simulink library "qrd_matrix_library"  (Simulink 8.7)
settings: Solver=ode45  StartTime=0.0  StopTime=10.0  RelTol=1e-3
values from neighbouring files (symbols this model uses):
  vectorization = 2    [qrd_test.m]
undefined symbols (not defined in the file or in its folder): AdvDSPBChannelOutDisplay, AdvDSPBDMemDisplay, Back_Substitution_instances, column_count, column_count_1, column_count_2, dpoly, dspba_ChannelInVis, dspba_ChannelOutVis, dspba_internal_get_channel_ports, evalAionMaskParam, latency, primtype, QRD_vectorization, recipsqrt, row, row_count, row_count_1, row_count_2, UseDontCare, value, x
libraries: DSPBAPrim x683, DSPBAControl x37, qrd_matrix_library x33, DSPBAVectorUtil x6, DSPBAVectorPrim x3
(part 3 of 8)

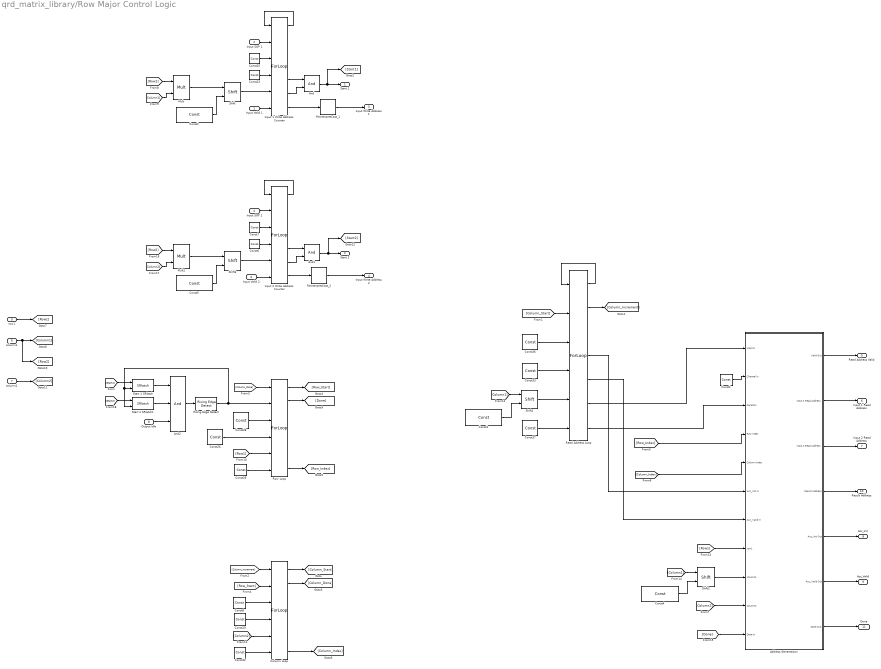
== system qrd_matrix_library/Row Major Control Logic ==
  Input Valid 1 : Inport
  Input SOP 1 : Inport  Port=2
  Input Valid 2 : Inport  Port=3
  Input SOP 2 : Inport  Port=4
  row1 : Inport  Port=5
  column1 : Inport  Port=6
  column2 : Inport  Port=7
  Output Idle : Inport  Port=8
  Address Generatioon : Subsystem
  And : DSPBAPrim/And  primtype=and  nInputs=2  nOutputs=1  omode=Inherit via internal rule  otype=sfix(16)  scale=2^-15  rndmethod=Unbiased  factor=1  satmethod=Symmetric  shift_vec=[0 1 2 -1]  value=0  inPortNames=[' '; ' '; ' '; ' '; ' '; ' '; ' '; ' '; ' '; ' '; ' '; ' '; ' '; ' '; ' '; ' '; ]  outPortNames=[' ']  dspbaimage=dspba_prim.jpg  text=fprintf('&');  style=Optimised  visibilities=8+2  version=20090407
  And1 : DSPBAPrim/And  primtype=and  nInputs=2  nOutputs=1  omode=Inherit via internal rule  otype=sfix(16)  scale=2^-15  rndmethod=Unbiased  factor=1  satmethod=Symmetric  shift_vec=[0 1 2 -1]  value=0  inPortNames=[' '; ' '; ' '; ' '; ' '; ' '; ' '; ' '; ' '; ' '; ' '; ' '; ' '; ' '; ' '; ' '; ]  outPortNames=[' ']  dspbaimage=dspba_prim.jpg  text=fprintf('&');  style=Optimised  visibilities=8+2  version=20090407
  And2 : DSPBAPrim/And  primtype=and  nInputs=3  nOutputs=1  omode=Inherit via internal rule  otype=sfix(16)  scale=2^-15  rndmethod=Unbiased  factor=1  satmethod=Symmetric  shift_vec=[0 1 2 -1]  value=0  inPortNames=[' '; ' '; ' '; ' '; ' '; ' '; ' '; ' '; ' '; ' '; ' '; ' '; ' '; ' '; ' '; ' '; ]  outPortNames=[' ']  dspbaimage=dspba_prim.jpg  text=fprintf('&');  style=Optimised  visibilities=8+2  version=20090407
  Column Loop : DSPBAPrim/ForLoop  looptest=<
  Const1 : DSPBAPrim/Const  primtype=const  nInputs=0  nOutputs=1  omode=Specify via dialog  otype=uint(8)  scale=1  rndmethod=Unbiased  factor=1  satmethod=Symmetric  shift_vec=[0 1 2 -1]  value=0  inPortNames=['+'; '+';]  outPortNames=[' ']  dspbaimage=dspba_prim.jpg  text=fprintf('%s', num2str(value));  style=Optimised  visibilities=8 + 1024  floatPrecision=float32_m23  version=20120820
  Const{2..5} (4 alike) : DSPBAPrim/Const  primtype=const  nInputs=0  nOutputs=1  omode=Inherit via internal rule  otype=uint(8)  scale=1  rndmethod=Unbiased  factor=1  satmethod=Symmetric  shift_vec=[0 1 2 -1]  value=nextpow2(vectorization)  inPortNames=['+'; '+';]  outPortNames=[' ']  dspbaimage=dspba_prim.jpg  text=fprintf('%s', num2str(value));  style=Optimised  visibilities=8 + 1024  floatPrecision=float32_m23  version=20120820
  Const{6,23,26,29,33,35,37} (7 alike) : DSPBAPrim/Const  primtype=const  nInputs=0  nOutputs=1  omode=Inherit via internal rule  otype=uint(8)  scale=1  rndmethod=Unbiased  factor=1  satmethod=Symmetric  shift_vec=[0 1 2 -1]  value=1  inPortNames=['+'; '+';]  outPortNames=[' ']  dspbaimage=dspba_prim.jpg  text=fprintf('%s', num2str(value));  style=Optimised  visibilities=8 + 1024  floatPrecision=float32_m23  version=20120820
  Const{7..8,25,28,36} (5 alike) : DSPBAPrim/Const  primtype=const  nInputs=0  nOutputs=1  omode=Inherit via internal rule  otype=uint(8)  scale=1  rndmethod=Unbiased  factor=1  satmethod=Symmetric  shift_vec=[0 1 2 -1]  value=0  inPortNames=['+'; '+';]  outPortNames=[' ']  dspbaimage=dspba_prim.jpg  text=fprintf('%s', num2str(value));  style=Optimised  visibilities=8 + 1024  floatPrecision=float32_m23  version=20120820
  Const32 : DSPBAPrim/Const  primtype=const  nInputs=0  nOutputs=1  omode=boolean  otype=uint(8)  scale=1  rndmethod=Unbiased  factor=1  satmethod=Symmetric  shift_vec=[0 1 2 -1]  value=1  inPortNames=['+'; '+';]  outPortNames=[' ']  dspbaimage=dspba_prim.jpg  text=fprintf('%s', num2str(value));  style=Optimised  visibilities=8 + 1024  floatPrecision=float32_m23  version=20120820
  Input 1 Write Address Counter : DSPBAPrim/ForLoop  looptest=<
  Input 2 Write Address Counter : DSPBAPrim/ForLoop  looptest=<
  Mult : DSPBAPrim/Mult  primtype=mult  nInputs=2  nOutputs=1  omode=Inherit via internal rule  otype=sfix(16)  scale=2^-15  rndmethod=Unbiased  factor=1  satmethod=Symmetric  shift_vec=[0 1 2 -1]  value=0  inPortNames=[' '; ' ';]  outPortNames=[' ']  dspbaimage=dspba_prim.jpg  text=fprintf('X');  style=Optimised  visibilities=8+2^18+2^19  floatPrecision=float32_m23  floatRounding=correct  advOptions=[]  version=20130115
  Mult1 : DSPBAPrim/Mult  primtype=mult  nInputs=2  nOutputs=1  omode=Inherit via internal rule  otype=sfix(16)  scale=2^-15  rndmethod=Unbiased  factor=1  satmethod=Symmetric  shift_vec=[0 1 2 -1]  value=0  inPortNames=[' '; ' ';]  outPortNames=[' ']  dspbaimage=dspba_prim.jpg  text=fprintf('X');  style=Optimised  visibilities=8+2^18+2^19  floatPrecision=float32_m23  floatRounding=correct  advOptions=[]  version=20130115
  Read Address Loop : DSPBAPrim/ForLoop  looptest=<
  ReinterpretCast_1 : DSPBAPrim/ReinterpretCast  primtype=reinterpret  nInputs=1  nOutputs=1  omode=Specify via dialog  otype=uint(nextpow2((row_count_1*column_count_1)/vectorization))  scale=1  rndmethod=Unbiased  factor=1  satmethod=Symmetric  shift_vec=[0 1 2 -1]  value=0  inPortNames=[' '; ' ';]  outPortNames=[' ']  dspbaimage=dspba_prim.jpg  text=fprintf('Reinterp\nCast', value);  style=Optimised  visibilities=8  floatPrecision=float32_m23  version=20120601
  ReinterpretCast_2 : DSPBAPrim/ReinterpretCast  primtype=reinterpret  nInputs=1  nOutputs=1  omode=Specify via dialog  otype=uint(nextpow2((row_count_2*column_count_2)/vectorization))  scale=1  rndmethod=Unbiased  factor=1  satmethod=Symmetric  shift_vec=[0 1 2 -1]  value=0  inPortNames=[' '; ' ';]  outPortNames=[' ']  dspbaimage=dspba_prim.jpg  text=fprintf('Reinterp\nCast', value);  style=Optimised  visibilities=8  floatPrecision=float32_m23  version=20120601
  Rising Edge Detect : qrd_matrix_library/matrix_multiplication/Rising Edge Detect
  Row Loop : DSPBAPrim/ForLoop  looptest=<
  Shift{,1..3} (4 alike) : DSPBAPrim/Shift  primtype=shift  nInputs=2  nOutputs=1  omode=Inherit via internal rule  otype=sfix(16)  scale=2^-15  rndmethod=Unbiased  factor=1  satmethod=Symmetric  shift_vec=[0 1 2 -1]  value=0  inPortNames=['a'; 'b';]  outPortNames=[' ']  dspbaimage=dspba_prim.jpg  text=fprintf('a >> b');  style=Optimised  visibilities=8  version=20090407
  Start 1 SRlatch : DSPBAControl/SRlatch
  Start 2 SRlatch1 : DSPBAControl/SRlatch
  Start 1 : Outport
  Start 2 : Outport  Port=2
  Input Write Address 1 : Outport  Port=3
  Input Write Address 2 : Outport  Port=4
  Read Address Valid : Outport  Port=5
  Input 1 Read Address : Outport  Port=6
  Input 2 Read Address : Outport  Port=7
  Acc_Init : Outport  Port=8
  Acc_Valid : Outport  Port=9
  Result Address : Outport  Port=10
  Done : Outport  Port=11
  wires:
  Address Generatioon/7(Done Out) -> Done/1
  [Done] -> Address Generatioon/11(Done In)
  [Column_Start] -> Read Address Loop/2
  Input SOP 1/1 -> Input 1 Write Address Counter/2
  Read Address Loop/2 -> [Column_Increment]
  Input 1 Write Address Counter/6 -> And/2
  Input 1 Write Address Counter/5 -> And/1
  Input 1 Write Address Counter/1 -> Input 1 Write Address Counter/1
  Input Valid 1/1 -> Input 1 Write Address Counter/6
  Shift2/1 -> Address Generatioon/9(column1)
  Const4/1 -> Shift2/2
  [Column1] -> Shift2/1
  [Row1] -> Address Generatioon/8(row1)
  Const3/1 -> Shift1/2
  [Column1] -> Shift1/1
  Const2/1 -> Shift/2
  Mult/1 -> Shift/1
  [Column1] -> Mult/2
  [Row1] -> Mult/1
  column1/1 -> [Row2], [Column1]
  row1/1 -> [Row1]
  Const1/1 -> Address Generatioon/2(Channel In)
  Address Generatioon/5(Acc_Init Out) -> Acc_Init/1
  Address Generatioon/6(Acc_Valid Out) -> Acc_Valid/1
  Read Address Loop/6 -> Address Generatioon/1(Valid In)
  Address Generatioon/4(Result Address) -> Result Address/1
  Address Generatioon/2(Input 1 Read Address) -> Input 1 Read Address/1
  Address Generatioon/3(Input 2 Read Address) -> Input 2 Read Address/1
  [Column_Index] -> Address Generatioon/5(Column Index)
  [Row_Index] -> Address Generatioon/4(Row Index)
  Read Address Loop/7 -> Address Generatioon/3(Iteration)
  Row Loop/2 -> [Done]
  Read Address Loop/5 -> Address Generatioon/7(Acc_Valid In)
  Read Address Loop/4 -> Address Generatioon/6(Acc_Init In)
  Address Generatioon/1(Valid Out) -> Read Address Valid/1
  Column Loop/7 -> [Column_Index]
  Const37/1 -> Read Address Loop/6
  Row Loop/1 -> [Row_Start]
  [Row_Start] -> Column Loop/2
  [Column_Done] -> Row Loop/1
  Column Loop/2 -> [Column_Done]
  [Column_Increment] -> Column Loop/1
  Column Loop/1 -> [Column_Start]
  Const35/1 -> Row Loop/6
  Const32/1 -> Column Loop/6
  Shift1/1 -> Read Address Loop/5
  Const33/1 -> Read Address Loop/4
  Const36/1 -> Read Address Loop/3
  Read Address Loop/1 -> Read Address Loop/1
  Row Loop/7 -> [Row_Index]
  Rising Edge Detect/1 -> Row Loop/2, Start 1 SRlatch/2, Start 2 SRlatch1/2
  Const29/1 -> Column Loop/4
  [Column2] -> Column Loop/5
  Const28/1 -> Row Loop/3
  Const26/1 -> Row Loop/4
  [Row1] -> Row Loop/5
  Input 1 Write Address Counter/7 -> ReinterpretCast_1/1
  Const25/1 -> Input 1 Write Address Counter/3
  Const23/1 -> Input 1 Write Address Counter/4
  Shift/1 -> Input 1 Write Address Counter/5
  column2/1 -> [Column2]
  Input SOP 2/1 -> Input 2 Write Address Counter/2
  Input 2 Write Address Counter/6 -> And1/2
  Input 2 Write Address Counter/5 -> And1/1
  Input 2 Write Address Counter/1 -> Input 2 Write Address Counter/1
  Input Valid 2/1 -> Input 2 Write Address Counter/6
  Const5/1 -> Shift3/2
  Mult1/1 -> Shift3/1
  [Column2] -> Mult1/2
  [Row2] -> Mult1/1
  Input 2 Write Address Counter/7 -> ReinterpretCast_2/1
  Const7/1 -> Input 2 Write Address Counter/3
  Const6/1 -> Input 2 Write Address Counter/4
  Shift3/1 -> Input 2 Write Address Counter/5
  And/1 -> [Start1], Start 1/1
  And1/1 -> [Start2], Start 2/1
  [Start1] -> Start 1 SRlatch/1
  [Start2] -> Start 2 SRlatch1/1
  And2/1 -> Rising Edge Detect/1
  Const8/1 -> Column Loop/3
  [Column2] -> Address Generatioon/10(column2)
  ReinterpretCast_1/1 -> Input Write Address 1/1
  ReinterpretCast_2/1 -> Input Write Address 2/1
  Output Idle/1 -> And2/3
  Start 1 SRlatch/1 -> And2/1
  Start 2 SRlatch1/1 -> And2/2

== system qrd_matrix_library/TappedDelay ==
  Data_In : Inport
  Mux : Mux  Inputs=2
  tap1 : DSPBAPrim/SampleDelay  primtype=sampdelay  nInputs=1  nOutputs=1  omode=Inherit via internal rule  otype=sfix(16)  scale=2^-15  rndmethod=Unbiased  factor=1  satmethod=Symmetric  shift_vec=[0 1 2 -1]  value=1  inPortNames=[' '; ' ';]  outPortNames=[' ']  dspbaimage=dspba_prim.jpg  text=dpoly(1, eye(1,value+1), 'z')  style=Optimised  visibilities=8 + 1024 + 2^17 + 2^18  flexible=off  slackgroup=0  augmented=0  version=20090407  advOptions=[]
  Data_Out : Outport
  wires:
  Data_In/1 -> Mux/2, tap1/1
  Mux/1 -> Data_Out/1
  tap1/1 -> Mux/1

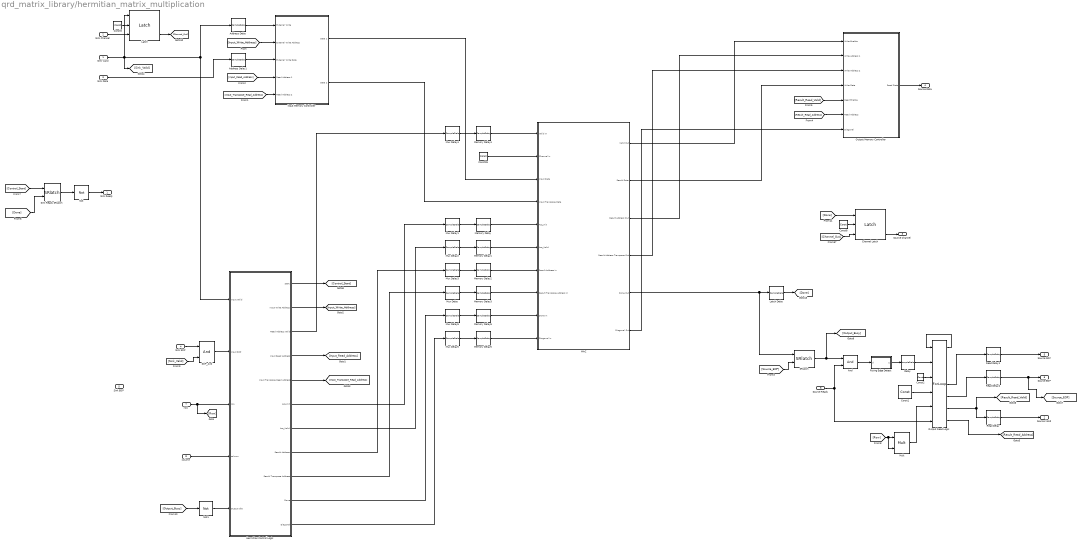
== system qrd_matrix_library/hermitian_matrix_multiplication ==
  Sink Valid : Inport
  Sink Channel : Inport  Port=2
  Sink Data : Inport  Port=3
  Sink SOP : Inport  Port=4
  Sink EOP : Inport  Port=5
  Source Ready : Inport  Port=6
  row : Inport  Port=7
  column : Inport  Port=8
  Address Delay : DSPBAPrim/SampleDelay  primtype=sampdelay  nInputs=1  nOutputs=1  omode=Inherit via internal rule  otype=sfix(16)  scale=2^-15  rndmethod=Unbiased  factor=1  satmethod=Symmetric  shift_vec=[0 1 2 -1]  value=1  inPortNames=[' '; ' ';]  outPortNames=[' ']  dspbaimage=dspba_prim.jpg  text=dpoly(1, eye(1,value+1), 'z')  style=Optimised  visibilities=8 + 1024 + 2^17 + 2^18  flexible=off  slackgroup=0  augmented=0  version=20090407  advOptions=[]
  Address Delay1 : DSPBAPrim/SampleDelay  primtype=sampdelay  nInputs=1  nOutputs=1  omode=Inherit via internal rule  otype=sfix(16)  scale=2^-15  rndmethod=Unbiased  factor=1  satmethod=Symmetric  shift_vec=[0 1 2 -1]  value=1  inPortNames=[' '; ' ';]  outPortNames=[' ']  dspbaimage=dspba_prim.jpg  text=dpoly(1, eye(1,value+1), 'z')  style=Optimised  visibilities=8 + 1024 + 2^17 + 2^18  flexible=off  slackgroup=0  augmented=0  version=20090407  advOptions=[]
  And : DSPBAPrim/And  primtype=and  nInputs=2  nOutputs=1  omode=Inherit via internal rule  otype=sfix(16)  scale=2^-15  rndmethod=Unbiased  factor=1  satmethod=Symmetric  shift_vec=[0 1 2 -1]  value=0  inPortNames=[' '; ' '; ' '; ' '; ' '; ' '; ' '; ' '; ' '; ' '; ' '; ' '; ' '; ' '; ' '; ' '; ]  outPortNames=[' ']  dspbaimage=dspba_prim.jpg  text=fprintf('&');  style=Optimised  visibilities=8+2  version=20090407
  Channel Latch : qrd_matrix_library/Latch
  Const1 : DSPBAPrim/Const  primtype=const  nInputs=0  nOutputs=1  omode=Inherit via internal rule  otype=uint(nextpow2(row*row))  scale=1  rndmethod=Unbiased  factor=1  satmethod=Symmetric  shift_vec=[0 1 2 -1]  value=1  inPortNames=['+'; '+';]  outPortNames=[' ']  dspbaimage=dspba_prim.jpg  text=fprintf('%s', num2str(value));  style=Optimised  visibilities=8 + 1024  floatPrecision=float32_m23  version=20120820
  Const2 : DSPBAPrim/Const  primtype=const  nInputs=0  nOutputs=1  omode=Specify via dialog  otype=uint(nextpow2(row_count*row_count))  scale=1  rndmethod=Unbiased  factor=1  satmethod=Symmetric  shift_vec=[0 1 2 -1]  value=0  inPortNames=['+'; '+';]  outPortNames=[' ']  dspbaimage=dspba_prim.jpg  text=fprintf('%s', num2str(value));  style=Optimised  visibilities=8 + 1024  floatPrecision=float32_m23  version=20120820
  Const26 : DSPBAPrim/Const  primtype=const  nInputs=0  nOutputs=1  omode=Specify via dialog  otype=uint(8)  scale=1  rndmethod=Unbiased  factor=1  satmethod=Symmetric  shift_vec=[0 1 2 -1]  value=0  inPortNames=['+'; '+';]  outPortNames=[' ']  dspbaimage=dspba_prim.jpg  text=fprintf('%s', num2str(value));  style=Optimised  visibilities=8 + 1024  floatPrecision=float32_m23  version=20120820
  Const6 : DSPBAPrim/Const  primtype=const  nInputs=0  nOutputs=1  omode=Specify via dialog  otype=uint(8)  scale=1  rndmethod=Unbiased  factor=1  satmethod=Symmetric  shift_vec=[0 1 2 -1]  value=0  inPortNames=['+'; '+';]  outPortNames=[' ']  dspbaimage=dspba_prim.jpg  text=fprintf('%s', num2str(value));  style=Optimised  visibilities=8 + 1024  floatPrecision=float32_m23  version=20120820
  Const8 : DSPBAPrim/Const  primtype=const  nInputs=0  nOutputs=1  omode=Specify via dialog  otype=uint(8)  scale=1  rndmethod=Unbiased  factor=1  satmethod=Symmetric  shift_vec=[0 1 2 -1]  value=0  inPortNames=['+'; '+';]  outPortNames=[' ']  dspbaimage=dspba_prim.jpg  text=fprintf('%s', num2str(value));  style=Optimised  visibilities=8 + 1024  floatPrecision=float32_m23  version=20120820
  Delay : DSPBAPrim/SampleDelay  primtype=sampdelay  nInputs=1  nOutputs=1  omode=Inherit via internal rule  otype=sfix(16)  scale=2^-15  rndmethod=Unbiased  factor=1  satmethod=Symmetric  shift_vec=[0 1 2 -1]  value=1  inPortNames=[' '; ' ';]  outPortNames=[' ']  dspbaimage=dspba_prim.jpg  text=dpoly(1, eye(1,value+1), 'z')  style=Optimised  visibilities=8 + 1024 + 2^17 + 2^18  flexible=off  slackgroup=0  augmented=0  version=20090407  advOptions=[]
  Hermitian Control Logic : Subsystem  BlockChoice=Hermitian Row Major Control Logic
      settings: AttributesFormatString=%<BlockChoice>  TemplateBlock=qrd_matrix_library/Hermitian Control Logic  MemberBlocks=Hermitian Column Major Control Logic,Hermitian Row Major Control Logic
  Input Memory Controller : Subsystem
  Latch : qrd_matrix_library/Latch
  Latch Delay : DSPBAPrim/SampleDelay  primtype=sampdelay  nInputs=1  nOutputs=1  omode=Inherit via internal rule  otype=sfix(16)  scale=2^-15  rndmethod=Unbiased  factor=1  satmethod=Symmetric  shift_vec=[0 1 2 -1]  value=1  inPortNames=[' '; ' ';]  outPortNames=[' ']  dspbaimage=dspba_prim.jpg  text=dpoly(1, eye(1,value+1), 'z')  style=Optimised  visibilities=8 + 1024 + 2^17 + 2^18  flexible=off  slackgroup=0  augmented=0  version=20090407  advOptions=[]
  MAC : Subsystem
  Memory Delay{,1..6} (7 alike) : DSPBAPrim/SampleDelay  primtype=sampdelay  nInputs=1  nOutputs=1  omode=Inherit via internal rule  otype=sfix(16)  scale=2^-15  rndmethod=Unbiased  factor=1  satmethod=Symmetric  shift_vec=[0 1 2 -1]  value=2  inPortNames=[' '; ' ';]  outPortNames=[' ']  dspbaimage=dspba_prim.jpg  text=dpoly(1, eye(1,value+1), 'z')  style=Optimised  visibilities=8 + 1024 + 2^17 + 2^18  flexible=off  slackgroup=0  augmented=0  version=20090407  advOptions=[]
  Mult : DSPBAPrim/Mult  primtype=mult  nInputs=2  nOutputs=1  omode=Inherit via internal rule  otype=sfix(16)  scale=2^-15  rndmethod=Unbiased  factor=1  satmethod=Symmetric  shift_vec=[0 1 2 -1]  value=0  inPortNames=[' '; ' ';]  outPortNames=[' ']  dspbaimage=dspba_prim.jpg  text=fprintf('X');  style=Optimised  visibilities=8+2^18+2^19  floatPrecision=float32_m23  floatRounding=correct  advOptions=[]  version=20130115
  Mux Delay{,1..6} (7 alike) : DSPBAPrim/SampleDelay  primtype=sampdelay  nInputs=1  nOutputs=1  omode=Inherit via internal rule  otype=sfix(16)  scale=2^-15  rndmethod=Unbiased  factor=1  satmethod=Symmetric  shift_vec=[0 1 2 -1]  value=1  inPortNames=[' '; ' ';]  outPortNames=[' ']  dspbaimage=dspba_prim.jpg  text=dpoly(1, eye(1,value+1), 'z')  style=Optimised  visibilities=8 + 1024 + 2^17 + 2^18  flexible=off  slackgroup=0  augmented=0  version=20090407  advOptions=[]
  Not : DSPBAPrim/Not  primtype=not  nInputs=1  nOutputs=1  omode=Inherit via internal rule  otype=sfix(16)  scale=2^-15  rndmethod=Unbiased  factor=1  satmethod=Symmetric  shift_vec=[0 1 2 -1]  value=0  inPortNames=[' '; ' ';]  outPortNames=[' ']  dspbaimage=dspba_prim.jpg  text=fprintf('~');  style=Optimised  visibilities=8  version=20090407
  Not1 : DSPBAPrim/Not  primtype=not  nInputs=1  nOutputs=1  omode=Inherit via internal rule  otype=sfix(16)  scale=2^-15  rndmethod=Unbiased  factor=1  satmethod=Symmetric  shift_vec=[0 1 2 -1]  value=0  inPortNames=[' '; ' ';]  outPortNames=[' ']  dspbaimage=dspba_prim.jpg  text=fprintf('~');  style=Optimised  visibilities=8  version=20090407
  Output Memory Controller : Subsystem
  Output Read Logic : DSPBAPrim/ForLoop  looptest=<
  Read Delay : DSPBAPrim/SampleDelay  primtype=sampdelay  nInputs=1  nOutputs=1  omode=Inherit via internal rule  otype=sfix(16)  scale=2^-15  rndmethod=Unbiased  factor=1  satmethod=Symmetric  shift_vec=[0 1 2 -1]  value=3  inPortNames=[' '; ' ';]  outPortNames=[' ']  dspbaimage=dspba_prim.jpg  text=dpoly(1, eye(1,value+1), 'z')  style=Optimised  visibilities=8 + 1024 + 2^17 + 2^18  flexible=off  slackgroup=0  augmented=0  version=20090407  advOptions=[]
  Read Delay1 : DSPBAPrim/SampleDelay  primtype=sampdelay  nInputs=1  nOutputs=1  omode=Inherit via internal rule  otype=sfix(16)  scale=2^-15  rndmethod=Unbiased  factor=1  satmethod=Symmetric  shift_vec=[0 1 2 -1]  value=3  inPortNames=[' '; ' ';]  outPortNames=[' ']  dspbaimage=dspba_prim.jpg  text=dpoly(1, eye(1,value+1), 'z')  style=Optimised  visibilities=8 + 1024 + 2^17 + 2^18  flexible=off  slackgroup=0  augmented=0  version=20090407  advOptions=[]
  Read Delay2 : DSPBAPrim/SampleDelay  primtype=sampdelay  nInputs=1  nOutputs=1  omode=Inherit via internal rule  otype=sfix(16)  scale=2^-15  rndmethod=Unbiased  factor=1  satmethod=Symmetric  shift_vec=[0 1 2 -1]  value=3  inPortNames=[' '; ' ';]  outPortNames=[' ']  dspbaimage=dspba_prim.jpg  text=dpoly(1, eye(1,value+1), 'z')  style=Optimised  visibilities=8 + 1024 + 2^17 + 2^18  flexible=off  slackgroup=0  augmented=0  version=20090407  advOptions=[]
  Rising Edge Detect : Subsystem  Opaque=on
      mask help:
      | The EdgeDetect component detects edges,
      | under the assumption that initial state
      | of the signal is 0 i.e. a 1 on the input
      | in the first cycle will be detected as
      | an edge.
      mask Help: helpview(dspba.GetHelp('EdgeDetect'));
      mask Display:
      | color('w');
      | image(imread('dspba_fft.jpg'));
      | port_label('input',1,'d');
      | port_label('output',1,'q');
      | text(0.4,0.5,sprintf('RED'));
  SOP_And : DSPBAPrim/And  primtype=and  nInputs=2  nOutputs=1  omode=Inherit via internal rule  otype=sfix(16)  scale=2^-15  rndmethod=Unbiased  factor=1  satmethod=Symmetric  shift_vec=[0 1 2 -1]  value=0  inPortNames=[' '; ' '; ' '; ' '; ' '; ' '; ' '; ' '; ' '; ' '; ' '; ' '; ' '; ' '; ' '; ' '; ]  outPortNames=[' ']  dspbaimage=dspba_prim.jpg  text=fprintf('&');  style=Optimised  visibilities=8+2  version=20090407
  SRlatch : DSPBAControl/SRlatch
  Sink Ready SRlatch : DSPBAControl/SRlatch
  Sink Ready : Outport
  Source Valid : Outport  Port=2
  Source Channel : Outport  Port=3
  Source Data : Outport  Port=4
  Source SOP : Outport  Port=5
  Source EOP : Outport  Port=6
  wires:
  Read Delay1/1 -> Source SOP/1
  Read Delay/1 -> Source Valid/1
  Mux Delay1/1 -> Memory Delay/1
  Memory Delay2/1 -> MAC/7(Result Address In)
  Memory Delay3/1 -> MAC/8(Result Transpose Address In)
  Output Memory Controller/1(Read Data) -> Source Data/1
  Address Delay/1 -> Input Memory Controller/1(External Write)
  Mux Delay/1 -> Memory Delay3/1
  Sink Data/1 -> Address Delay1/1
  Memory Delay/1 -> MAC/5(Acc_Init)
  Hermitian Control Logic/10(Done) -> Mux Delay6/1
  MAC/3(Result Address Out) -> Output Memory Controller/2(Write Address 1)
  Mux Delay3/1 -> Memory Delay2/1
  MAC/4(Result Address Transpose Out) -> Output Memory Controller/3(Write Address 2)
  MAC/2(Result Data) -> Output Memory Controller/4(Write Data)
  Mux Delay4/1 -> Memory Delay4/1
  Hermitian Control Logic/2(Input Write Address) -> [Input_Write_Address]
  Address Delay1/1 -> Input Memory Controller/3(External Write Data)
  Source Ready/1 -> Output Read Logic/6, And/2
  [Input_Write_Address] -> Input Memory Controller/2(External Write Address)
  Memory Delay4/1 -> MAC/1(Valid In)
  Read Delay2/1 -> [Source_EOP], Source EOP/1
  Mux Delay2/1 -> Memory Delay1/1
  MAC/1(Valid Out) -> Output Memory Controller/1(Write Enable)
  Hermitian Control Logic/4(Input Read Address) -> [Input_Read_Address]
  [Result_Read_Address] -> Output Memory Controller/6(Read Address)
  Rising Edge Detect/1(q) -> Delay/1
  Sink SOP/1 -> SOP_And/1
  Hermitian Control Logic/6(Acc_Init) -> Mux Delay1/1
  Const26/1 -> MAC/2(Channel In)
  Hermitian Control Logic/8(Result Address) -> Mux Delay3/1
  [Input_Read_Address] -> Input Memory Controller/4(Read Address 1)
  [Input_Transpose_Read_Address] -> Input Memory Controller/5(Read Address 2)
  And/1 -> Rising Edge Detect/1(d)
  Memory Delay1/1 -> MAC/6(Acc_Valid)
  Input Memory Controller/2(Data 2) -> MAC/4(Input Transpose Data)
  Input Memory Controller/1(Data 1) -> MAC/3(Input Data)
  Hermitian Control Logic/9(Result Transpose Address) -> Mux Delay/1
  Sink Valid/1 -> [Sink_Valid], Hermitian Control Logic/1(Input Valid), Address Delay/1, Latch/1
  Hermitian Control Logic/5(Input Transpose Read Address) -> [Input_Transpose_Read_Address]
  Hermitian Control Logic/7(Acc_Valid) -> Mux Delay2/1
  Hermitian Control Logic/3(Read Address Valid) -> Mux Delay4/1
  Delay/1 -> Output Read Logic/2
  [Result_Read_Valid] -> Output Memory Controller/5(Read Enable)
  Output Read Logic/6 -> Read Delay/1, [Result_Read_Valid]
  Output Read Logic/7 -> [Result_Read_Address]
  Output Read Logic/4 -> Read Delay1/1
  Output Read Logic/5 -> Read Delay2/1
  Mult/1 -> Output Read Logic/5
  Const1/1 -> Output Read Logic/4
  Const2/1 -> Output Read Logic/3
  Output Read Logic/1 -> Output Read Logic/1
  Hermitian Control Logic/11(Diagonal) -> Mux Delay5/1
  MAC/6(Diagonal Out) -> Output Memory Controller/7(Diagonal)
  Mux Delay5/1 -> Memory Delay5/1
  Memory Delay5/1 -> MAC/10(Diagonal In)
  Mux Delay6/1 -> Memory Delay6/1
  Memory Delay6/1 -> MAC/9(Done In)
  [Source_EOP] -> SRlatch/2
  row/1 -> Hermitian Control Logic/3(row), [Row]
  column/1 -> Hermitian Control Logic/4(column)
  Not/1 -> Sink Ready/1
  [Done] -> Sink Ready SRlatch/2
  [Row] -> Mult/2, Mult/1
  Sink Channel/1 -> Latch/3
  Const6/1 -> Latch/2
  Latch/3 -> [Channel_Out]
  Sink Ready SRlatch/1 -> Not/1
  [Sink_Valid] -> SOP_And/2
  SOP_And/1 -> Hermitian Control Logic/2(Input SOP)
  Hermitian Control Logic/1(Start) -> [Control_Start]
  [Control_Start] -> Sink Ready SRlatch/1
  SRlatch/1 -> [Output_Busy], And/1
  MAC/5(Done Out) -> SRlatch/1, Latch Delay/1
  Latch Delay/1 -> [Done]
  Not1/1 -> Hermitian Control Logic/5(Output Idle)
  [Output_Busy] -> Not1/1
  [Channel_Out] -> Channel Latch/3
  Const8/1 -> Channel Latch/2
  [Done] -> Channel Latch/1
  Channel Latch/3 -> Source Channel/1

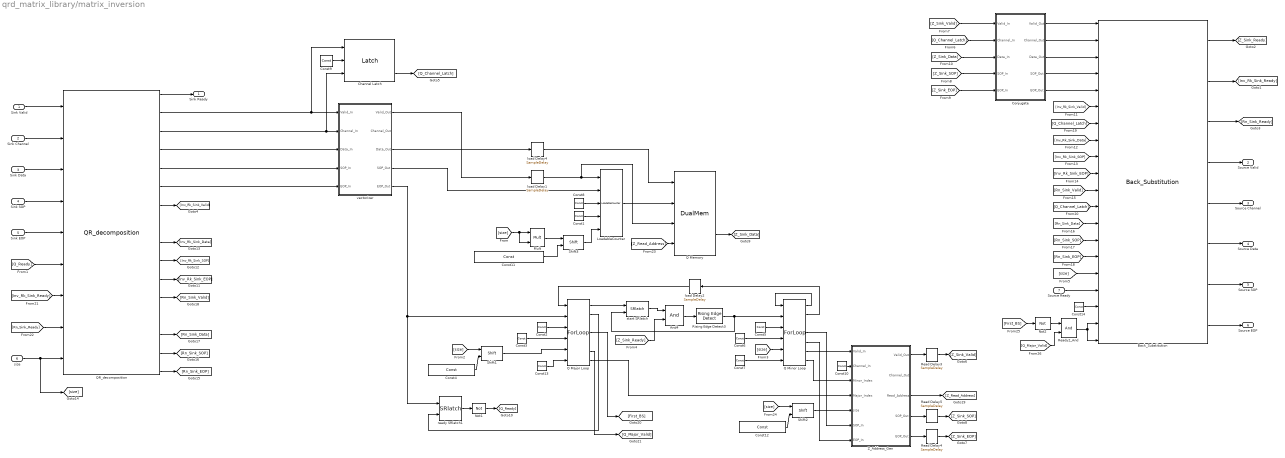
== system qrd_matrix_library/matrix_inversion ==
  Sink Valid : Inport
  Sink Channel : Inport  Port=2
  Sink Data : Inport  Port=3
  Sink SOP : Inport  Port=4
  Sink EOP : Inport  Port=5
  size : Inport  Port=6
  Source Ready : Inport  Port=7
  And4 : DSPBAPrim/And  primtype=and  nInputs=2  nOutputs=1  omode=Inherit via internal rule  otype=sfix(16)  scale=2^-15  rndmethod=Unbiased  factor=1  satmethod=Symmetric  shift_vec=[0 1 2 -1]  value=0  inPortNames=[' '; ' '; ' '; ' '; ' '; ' '; ' '; ' '; ' '; ' '; ' '; ' '; ' '; ' '; ' '; ' '; ]  outPortNames=[' ']  dspbaimage=dspba_prim.jpg  text=fprintf('&');  style=Optimised  visibilities=8+2  version=20090407
  Back_Substitution : qrd_matrix_library/Back_Substitution  size=size  instances=4
  Channel Latch : qrd_matrix_library/Latch
  Conjugate : Subsystem
  Const1 : DSPBAPrim/Const  primtype=const  nInputs=0  nOutputs=1  omode=Inherit via internal rule  otype=uint(8)  scale=1  rndmethod=Unbiased  factor=1  satmethod=Symmetric  shift_vec=[0 1 2 -1]  value=1  inPortNames=['+'; '+';]  outPortNames=[' ']  dspbaimage=dspba_prim.jpg  text=fprintf('%s', num2str(value));  style=Optimised  visibilities=8 + 1024  floatPrecision=float32_m23  version=20120820
  Const10 : DSPBAPrim/Const  primtype=const  nInputs=0  nOutputs=1  omode=Specify via dialog  otype=uint(8)  scale=1  rndmethod=Unbiased  factor=1  satmethod=Symmetric  shift_vec=[0 1 2 -1]  value=0  inPortNames=['+'; '+';]  outPortNames=[' ']  dspbaimage=dspba_prim.jpg  text=fprintf('%s', num2str(value));  style=Optimised  visibilities=8 + 1024  floatPrecision=float32_m23  version=20120820
  Const11 : DSPBAPrim/Const  primtype=const  nInputs=0  nOutputs=1  omode=Inherit via internal rule  otype=uint(8)  scale=1  rndmethod=Unbiased  factor=1  satmethod=Symmetric  shift_vec=[0 1 2 -1]  value=nextpow2(Back_Substitution_instances)  inPortNames=['+'; '+';]  outPortNames=[' ']  dspbaimage=dspba_prim.jpg  text=fprintf('%s', num2str(value));  style=Optimised  visibilities=8 + 1024  floatPrecision=float32_m23  version=20120820
  Const12 : DSPBAPrim/Const  primtype=const  nInputs=0  nOutputs=1  omode=Inherit via internal rule  otype=uint(8)  scale=1  rndmethod=Unbiased  factor=1  satmethod=Symmetric  shift_vec=[0 1 2 -1]  value=nextpow2(Back_Substitution_instances)  inPortNames=['+'; '+';]  outPortNames=[' ']  dspbaimage=dspba_prim.jpg  text=fprintf('%s', num2str(value));  style=Optimised  visibilities=8 + 1024  floatPrecision=float32_m23  version=20120820
  Const13 : DSPBAPrim/Const  primtype=const  nInputs=0  nOutputs=1  omode=boolean  otype=uint(8)  scale=1  rndmethod=Unbiased  factor=1  satmethod=Symmetric  shift_vec=[0 1 2 -1]  value=1  inPortNames=['+'; '+';]  outPortNames=[' ']  dspbaimage=dspba_prim.jpg  text=fprintf('%s', num2str(value));  style=Optimised  visibilities=8 + 1024  floatPrecision=float32_m23  version=20120820
  Const14 : DSPBAPrim/Const  primtype=const  nInputs=0  nOutputs=1  omode=boolean  otype=uint(8)  scale=1  rndmethod=Unbiased  factor=1  satmethod=Symmetric  shift_vec=[0 1 2 -1]  value=0  inPortNames=['+'; '+';]  outPortNames=[' ']  dspbaimage=dspba_prim.jpg  text=fprintf('%s', num2str(value));  style=Optimised  visibilities=8 + 1024  floatPrecision=float32_m23  version=20120820
  Const2 : DSPBAPrim/Const  primtype=const  nInputs=0  nOutputs=1  omode=Inherit via internal rule  otype=uint(8)  scale=1  rndmethod=Unbiased  factor=1  satmethod=Symmetric  shift_vec=[0 1 2 -1]  value=0  inPortNames=['+'; '+';]  outPortNames=[' ']  dspbaimage=dspba_prim.jpg  text=fprintf('%s', num2str(value));  style=Optimised  visibilities=8 + 1024  floatPrecision=float32_m23  version=20120820
  Const3 : DSPBAPrim/Const  primtype=const  nInputs=0  nOutputs=1  omode=Inherit via internal rule  otype=uint(8)  scale=1  rndmethod=Unbiased  factor=1  satmethod=Symmetric  shift_vec=[0 1 2 -1]  value=1  inPortNames=['+'; '+';]  outPortNames=[' ']  dspbaimage=dspba_prim.jpg  text=fprintf('%s', num2str(value));  style=Optimised  visibilities=8 + 1024  floatPrecision=float32_m23  version=20120820
  Const4 : DSPBAPrim/Const  primtype=const  nInputs=0  nOutputs=1  omode=Inherit via internal rule  otype=uint(8)  scale=1  rndmethod=Unbiased  factor=1  satmethod=Symmetric  shift_vec=[0 1 2 -1]  value=nextpow2(Back_Substitution_instances)  inPortNames=['+'; '+';]  outPortNames=[' ']  dspbaimage=dspba_prim.jpg  text=fprintf('%s', num2str(value));  style=Optimised  visibilities=8 + 1024  floatPrecision=float32_m23  version=20120820
  Const5 : DSPBAPrim/Const  primtype=const  nInputs=0  nOutputs=1  omode=Inherit via internal rule  otype=uint(8)  scale=1  rndmethod=Unbiased  factor=1  satmethod=Symmetric  shift_vec=[0 1 2 -1]  value=0  inPortNames=['+'; '+';]  outPortNames=[' ']  dspbaimage=dspba_prim.jpg  text=fprintf('%s', num2str(value));  style=Optimised  visibilities=8 + 1024  floatPrecision=float32_m23  version=20120820
  Const6 : DSPBAPrim/Const  primtype=const  nInputs=0  nOutputs=1  omode=Inherit via internal rule  otype=uint(8)  scale=1  rndmethod=Unbiased  factor=1  satmethod=Symmetric  shift_vec=[0 1 2 -1]  value=1  inPortNames=['+'; '+';]  outPortNames=[' ']  dspbaimage=dspba_prim.jpg  text=fprintf('%s', num2str(value));  style=Optimised  visibilities=8 + 1024  floatPrecision=float32_m23  version=20120820
  Const7 : DSPBAPrim/Const  primtype=const  nInputs=0  nOutputs=1  omode=boolean  otype=uint(8)  scale=1  rndmethod=Unbiased  factor=1  satmethod=Symmetric  shift_vec=[0 1 2 -1]  value=1  inPortNames=['+'; '+';]  outPortNames=[' ']  dspbaimage=dspba_prim.jpg  text=fprintf('%s', num2str(value));  style=Optimised  visibilities=8 + 1024  floatPrecision=float32_m23  version=20120820
  Const8 : DSPBAPrim/Const  primtype=const  nInputs=0  nOutputs=1  omode=Inherit via internal rule  otype=uint(8)  scale=1  rndmethod=Unbiased  factor=1  satmethod=Symmetric  shift_vec=[0 1 2 -1]  value=0  inPortNames=['+'; '+';]  outPortNames=[' ']  dspbaimage=dspba_prim.jpg  text=fprintf('%s', num2str(value));  style=Optimised  visibilities=8 + 1024  floatPrecision=float32_m23  version=20120820
  Const9 : DSPBAPrim/Const  primtype=const  nInputs=0  nOutputs=1  omode=Specify via dialog  otype=uint(8)  scale=1  rndmethod=Unbiased  factor=1  satmethod=Symmetric  shift_vec=[0 1 2 -1]  value=0  inPortNames=['+'; '+';]  outPortNames=[' ']  dspbaimage=dspba_prim.jpg  text=fprintf('%s', num2str(value));  style=Optimised  visibilities=8 + 1024  floatPrecision=float32_m23  version=20120820
  LoadableCounter : DSPBAPrim/LoadableCounter  primtype=loadablecounter  nInputs=5  nOutputs=1  omode=Specify via dialog  otype=uint(nextpow2(size*size/Back_Substitution_instances))  scale=1  rndmethod=Unbiased  factor=1  satmethod=Symmetric  shift_vec=[0 1 2 -1]  value=[0 (size*size/Back_Substitution_instances) 1]  inPortNames=['en';'ld';'i ';'s ';'m ']  outPortNames=[' ']  dspbaimage=dspba_prim.jpg  text=fprintf('loadable\ncounter\n[%d %d %d]', value(1), value(2), value(3));  style=Optimised  visibilities=8 + 1024  version=20090407
  Mult : DSPBAPrim/Mult  primtype=mult  nInputs=2  nOutputs=1  omode=Inherit via internal rule  otype=sfix(16)  scale=2^-15  rndmethod=Unbiased  factor=1  satmethod=Symmetric  shift_vec=[0 1 2 -1]  value=0  inPortNames=[' '; ' ';]  outPortNames=[' ']  dspbaimage=dspba_prim.jpg  text=fprintf('X');  style=Optimised  visibilities=8+2^18+2^19  floatPrecision=float32_m23  floatRounding=correct  advOptions=[]  version=20130115
  Not1 : DSPBAPrim/Not  primtype=not  nInputs=1  nOutputs=1  omode=Inherit via internal rule  otype=sfix(16)  scale=2^-15  rndmethod=Unbiased  factor=1  satmethod=Symmetric  shift_vec=[0 1 2 -1]  value=0  inPortNames=[' '; ' ';]  outPortNames=[' ']  dspbaimage=dspba_prim.jpg  text=fprintf('~');  style=Optimised  visibilities=8  version=20090407
  Not2 : DSPBAPrim/Not  primtype=not  nInputs=1  nOutputs=1  omode=Inherit via internal rule  otype=sfix(16)  scale=2^-15  rndmethod=Unbiased  factor=1  satmethod=Symmetric  shift_vec=[0 1 2 -1]  value=0  inPortNames=[' '; ' ';]  outPortNames=[' ']  dspbaimage=dspba_prim.jpg  text=fprintf('~');  style=Optimised  visibilities=8  version=20090407
  Q Major Loop : DSPBAPrim/ForLoop  looptest=<
  Q Memory : DSPBAPrim/DualMem  primtype=dualmem  nInputs=4  nOutputs=2  omode=Inherit via internal rule  otype=sfix(16)  scale=2^-15  rndmethod=Unbiased  factor=1  satmethod=Symmetric  shift_vec=[0 1 2 -1]  value=complex(zeros(size*size/Back_Substitution_instances,Back_Substitution_instances),zeros(size*size/Back_Substitution_instances,Back_Substitution_instances))  inPortNames=['d1'; 'a1'; 'w1'; 'a2']  outPortNames=['q1'; 'q2']  dspbaimage=dspba_prim.jpg  text=fprintf('dmem%s',AdvDSPBDMemDisplay(UseDontCare));  style=Optimised  visibilities=8 + 1024 + 2^17 + 2^18  UseDontCare=on  TwinWritePorts=off  version=20141001
  Q Minor Loop : DSPBAPrim/ForLoop  looptest=<
  QR_decomposition : qrd_matrix_library/QR_decomposition  size=size  vectorization=QRD_vectorization
  Read Delay3 : DSPBAPrim/SampleDelay  primtype=sampdelay  nInputs=1  nOutputs=1  omode=Inherit via internal rule  otype=sfix(16)  scale=2^-15  rndmethod=Unbiased  factor=1  satmethod=Symmetric  shift_vec=[0 1 2 -1]  value=2  inPortNames=[' '; ' ';]  outPortNames=[' ']  dspbaimage=dspba_prim.jpg  text=dpoly(1, eye(1,value+1), 'z')  style=Optimised  visibilities=8 + 1024 + 2^17 + 2^18  flexible=off  slackgroup=0  augmented=0  version=20090407  advOptions=[]
  Read Delay4 : DSPBAPrim/SampleDelay  primtype=sampdelay  nInputs=1  nOutputs=1  omode=Inherit via internal rule  otype=sfix(16)  scale=2^-15  rndmethod=Unbiased  factor=1  satmethod=Symmetric  shift_vec=[0 1 2 -1]  value=2  inPortNames=[' '; ' ';]  outPortNames=[' ']  dspbaimage=dspba_prim.jpg  text=dpoly(1, eye(1,value+1), 'z')  style=Optimised  visibilities=8 + 1024 + 2^17 + 2^18  flexible=off  slackgroup=0  augmented=0  version=20090407  advOptions=[]
  Read Delay5 : DSPBAPrim/SampleDelay  primtype=sampdelay  nInputs=1  nOutputs=1  omode=Inherit via internal rule  otype=sfix(16)  scale=2^-15  rndmethod=Unbiased  factor=1  satmethod=Symmetric  shift_vec=[0 1 2 -1]  value=2  inPortNames=[' '; ' ';]  outPortNames=[' ']  dspbaimage=dspba_prim.jpg  text=dpoly(1, eye(1,value+1), 'z')  style=Optimised  visibilities=8 + 1024 + 2^17 + 2^18  flexible=off  slackgroup=0  augmented=0  version=20090407  advOptions=[]
  Ready2_And : DSPBAPrim/And  primtype=and  nInputs=2  nOutputs=1  omode=Inherit via internal rule  otype=sfix(16)  scale=2^-15  rndmethod=Unbiased  factor=1  satmethod=Symmetric  shift_vec=[0 1 2 -1]  value=0  inPortNames=[' '; ' '; ' '; ' '; ' '; ' '; ' '; ' '; ' '; ' '; ' '; ' '; ' '; ' '; ' '; ' '; ]  outPortNames=[' ']  dspbaimage=dspba_prim.jpg  text=fprintf('&');  style=Optimised  visibilities=8+2  version=20090407
  Rising Edge Detect3 : qrd_matrix_library/hermitian_matrix_multiplication/Rising Edge Detect
  Shift1 : DSPBAPrim/Shift  primtype=shift  nInputs=2  nOutputs=1  omode=Inherit via internal rule  otype=sfix(16)  scale=2^-15  rndmethod=Unbiased  factor=1  satmethod=Symmetric  shift_vec=[0 1 2 -1]  value=0  inPortNames=['a'; 'b';]  outPortNames=[' ']  dspbaimage=dspba_prim.jpg  text=fprintf('a >> b');  style=Optimised  visibilities=8  version=20090407
  Shift2 : DSPBAPrim/Shift  primtype=shift  nInputs=2  nOutputs=1  omode=Inherit via internal rule  otype=sfix(16)  scale=2^-15  rndmethod=Unbiased  factor=1  satmethod=Symmetric  shift_vec=[0 1 2 -1]  value=0  inPortNames=['a'; 'b';]  outPortNames=[' ']  dspbaimage=dspba_prim.jpg  text=fprintf('a >> b');  style=Optimised  visibilities=8  version=20090407
  Shift3 : DSPBAPrim/Shift  primtype=shift  nInputs=2  nOutputs=1  omode=Inherit via internal rule  otype=sfix(16)  scale=2^-15  rndmethod=Unbiased  factor=1  satmethod=Symmetric  shift_vec=[0 1 2 -1]  value=0  inPortNames=['a'; 'b';]  outPortNames=[' ']  dspbaimage=dspba_prim.jpg  text=fprintf('a >> b');  style=Optimised  visibilities=8  version=20090407
  Z_Address_Gen : Subsystem
  load Delay1 : DSPBAPrim/SampleDelay  primtype=sampdelay  nInputs=1  nOutputs=1  omode=Inherit via internal rule  otype=sfix(16)  scale=2^-15  rndmethod=Unbiased  factor=1  satmethod=Symmetric  shift_vec=[0 1 2 -1]  value=1  inPortNames=[' '; ' ';]  outPortNames=[' ']  dspbaimage=dspba_prim.jpg  text=dpoly(1, eye(1,value+1), 'z')  style=Optimised  visibilities=8 + 1024 + 2^17 + 2^18  flexible=off  slackgroup=0  augmented=0  version=20090407  advOptions=[]
  load Delay2 : DSPBAPrim/SampleDelay  primtype=sampdelay  nInputs=1  nOutputs=1  omode=Inherit via internal rule  otype=sfix(16)  scale=2^-15  rndmethod=Unbiased  factor=1  satmethod=Symmetric  shift_vec=[0 1 2 -1]  value=50  inPortNames=[' '; ' ';]  outPortNames=[' ']  dspbaimage=dspba_prim.jpg  text=dpoly(1, eye(1,value+1), 'z')  style=Optimised  visibilities=8 + 1024 + 2^17 + 2^18  flexible=off  slackgroup=0  augmented=0  version=20090407  advOptions=[]
  load Delay4 : DSPBAPrim/SampleDelay  primtype=sampdelay  nInputs=1  nOutputs=1  omode=Inherit via internal rule  otype=sfix(16)  scale=2^-15  rndmethod=Unbiased  factor=1  satmethod=Symmetric  shift_vec=[0 1 2 -1]  value=1  inPortNames=[' '; ' ';]  outPortNames=[' ']  dspbaimage=dspba_prim.jpg  text=dpoly(1, eye(1,value+1), 'z')  style=Optimised  visibilities=8 + 1024 + 2^17 + 2^18  flexible=off  slackgroup=0  augmented=0  version=20090407  advOptions=[]
  ready SRlatch1 : DSPBAControl/SRlatch
  start SRlatch : DSPBAControl/SRlatch
  vectorizer : Subsystem
  Sink Ready : Outport
  Source Valid : Outport  Port=2
  Source Channel : Outport  Port=3
  Source Data : Outport  Port=4
  Source SOP : Outport  Port=5
  Source EOP : Outport  Port=6
  wires:
  Sink Valid/1 -> QR_decomposition/1
  Sink Channel/1 -> QR_decomposition/2
  Sink SOP/1 -> QR_decomposition/4
  Sink EOP/1 -> QR_decomposition/5
  Sink Data/1 -> QR_decomposition/3
  [Q_Ready] -> QR_decomposition/6
  size/1 -> QR_decomposition/9, [size]
  Back_Substitution/1 -> [Z_Sink_Ready]
  Back_Substitution/4 -> Source Valid/1
  Back_Substitution/5 -> Source Channel/1
  Back_Substitution/6 -> Source Data/1
  Back_Substitution/7 -> Source SOP/1
  Back_Substitution/8 -> Source EOP/1
  QR_decomposition/1 -> Sink Ready/1
  Back_Substitution/3 -> [Rn_Sink_Ready]
  Back_Substitution/2 -> [Inv_Rk_Sink_Ready]
  vectorizer/4(SOP_Out) -> LoadableCounter/2
  Shift3/1 -> LoadableCounter/5
  Const1/1 -> LoadableCounter/4
  Const8/1 -> LoadableCounter/3
  [size] -> Mult/2, Mult/1
  LoadableCounter/1 -> Q Memory/2
  load Delay4/1 -> Q Memory/1
  load Delay1/1 -> Q Memory/3, LoadableCounter/1
  Const2/1 -> Q Major Loop/3
  Const3/1 -> Q Major Loop/4
  [size] -> Shift1/1
  Const13/1 -> Q Major Loop/6
  Q Minor Loop/1 -> Q Minor Loop/1
  Q Minor Loop/2 -> load Delay2/1
  Const5/1 -> Q Minor Loop/3
  Const6/1 -> Q Minor Loop/4
  Const7/1 -> Q Minor Loop/6
  [size] -> Q Minor Loop/5
  load Delay2/1 -> Q Major Loop/1
  Q Minor Loop/7 -> Z_Address_Gen/3(Minor_Index)
  [size] -> Back_Substitution/16
  Source Ready/1 -> Back_Substitution/17
  QR_decomposition/5 -> vectorizer/4(SOP_In)
  QR_decomposition/2 -> Channel Latch/1, vectorizer/1(Valid_In)
  QR_decomposition/3 -> Channel Latch/3, vectorizer/2(Channel_In)
  QR_decomposition/4 -> vectorizer/3(Data_In)
  QR_decomposition/6 -> vectorizer/5(EOP_In)
  vectorizer/3(Data_Out) -> load Delay4/1
  vectorizer/1(Valid_Out) -> load Delay1/1
  Const9/1 -> Channel Latch/2
  Channel Latch/3 -> [Q_Channel_Latch]
  Shift1/1 -> Q Major Loop/5
  Const4/1 -> Shift1/2
  Read Delay3/1 -> [Z_Sink_Valid]
  Read Delay4/1 -> [Z_Sink_EOP]
  Q Minor Loop/5 -> Z_Address_Gen/7(EOP_In)
  Read Delay5/1 -> [Z_Sink_SOP]
  Q Minor Loop/4 -> Z_Address_Gen/6(SOP_In)
  Q Memory/2 -> [Z_Sink_Data]
  Mult/1 -> Shift3/1
  Const11/1 -> Shift3/2
  [Z_Sink_Ready] -> And4/2
  And4/1 -> Rising Edge Detect3/1
  Q Major Loop/2 -> ready SRlatch1/2
  Not1/1 -> [Q_Ready]
  ready SRlatch1/1 -> Not1/1
  QR_decomposition/7 -> [Inv_Rk_Sink_Valid]
  QR_decomposition/11 -> [Inv_Rk_Sink_EOP]
  QR_decomposition/10 -> [Inv_Rk_Sink_SOP]
  QR_decomposition/9 -> [Inv_Rk_Sink_Data]
  QR_decomposition/15 -> [Rn_Sink_SOP]
  QR_decomposition/16 -> [Rn_Sink_EOP]
  QR_decomposition/14 -> [Rn_Sink_Data]
  QR_decomposition/12 -> [Rn_Sink_Valid]
  [Inv_Rk_Sink_Valid] -> Back_Substitution/6
  [Q_Channel_Latch] -> Back_Substitution/7
  [Inv_Rk_Sink_Data] -> Back_Substitution/8
  [Inv_Rk_Sink_SOP] -> Back_Substitution/9
  [Rn_Sink_Valid] -> Back_Substitution/11
  [Inv_Rk_Sink_EOP] -> Back_Substitution/10
  [Q_Channel_Latch] -> Back_Substitution/12
  [Rn_Sink_Data] -> Back_Substitution/13
  [Rn_Sink_SOP] -> Back_Substitution/14
  [Rn_Sink_EOP] -> Back_Substitution/15
  [Inv_Rk_Sink_Ready] -> QR_decomposition/7
  [Rn_Sink_Ready] -> QR_decomposition/8
  Q Minor Loop/6 -> Z_Address_Gen/1(Valid_In)
  Const10/1 -> Z_Address_Gen/2(Channel_In)
  Z_Address_Gen/5(EOP_Out) -> Read Delay4/1
  Z_Address_Gen/4(SOP_Out) -> Read Delay5/1
  Z_Address_Gen/1(Valid_Out) -> Read Delay3/1
  Q Major Loop/7 -> Z_Address_Gen/4(Major_Index)
  Z_Address_Gen/3(Read_Address) -> [Z_Read_Address]
  [Z_Read_Address] -> Q Memory/4
  [size] -> Shift2/1
  Const12/1 -> Shift2/2
  Shift2/1 -> Z_Address_Gen/5(size)
  Conjugate/1(Valid_Out) -> Back_Substitution/1
  Conjugate/2(Channel_Out) -> Back_Substitution/2
  Conjugate/3(Data_Out) -> Back_Substitution/3
  Conjugate/4(SOP_Out) -> Back_Substitution/4
  Conjugate/5(EOP_Out) -> Back_Substitution/5
  [Q_Channel_Latch] -> Conjugate/2(Channel_In)
  [Z_Sink_Valid] -> Conjugate/1(Valid_In)
  [Z_Sink_Data] -> Conjugate/3(Data_In)
  [Z_Sink_SOP] -> Conjugate/4(SOP_In)
  [Z_Sink_EOP] -> Conjugate/5(EOP_In)
  start SRlatch/1 -> And4/1
  vectorizer/5(EOP_Out) -> Q Major Loop/2, ready SRlatch1/1
  Q Major Loop/1 -> start SRlatch/1
  Rising Edge Detect3/1 -> start SRlatch/2, Q Minor Loop/2
  Const14/1 -> Back_Substitution/18
  Q Major Loop/4 -> [First_BS]
  [First_BS] -> Not2/1
  Not2/1 -> Ready2_And/1
  Ready2_And/1 -> Back_Substitution/20, Back_Substitution/19
  Q Major Loop/6 -> [Q_Major_Valid]
  [Q_Major_Valid] -> Ready2_And/2
